simulink model "ddm"  (R2021a)
settings: Solver=ode4  StartTime=0.0  StopTime=2  FixedStep=0.01  RelTol=1e-3
InitFcn:
  | d = 1;
  | k = 1;
  | m = 1;
  | s0 = 1;
  | v0 = 1;
settings Model: Creator=ceanb  LastModifiedBy=peter

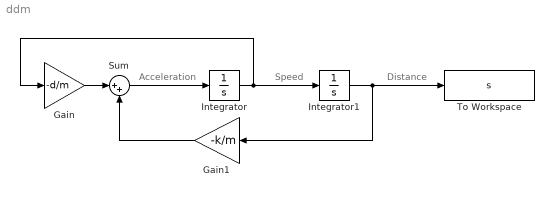
== system ddm ==
  note: Acceleration
  note: Speed
  note: Distance
  Gain : Gain  Gain=-d/m
  Gain1 : Gain  Gain=-k/m
  Integrator : Integrator  InitialCondition=v0
  Integrator1 : Integrator  InitialCondition=s0
  Sum : Sum  Inputs=|++
  To Workspace : ToWorkspace  VariableName=s  SampleTime=-1
      settings: Save2DSignal=2-D array (concatenate along first dimension)
  wires:
  Integrator/1 -> Gain/1, Integrator1/1
  Sum/1 -> Integrator/1
  Gain/1 -> Sum/1
  Integrator1/1 -> To Workspace/1, Gain1/1
  Gain1/1 -> Sum/2
